simulink model "SOLAR20KW10KW_MOTOR2SWitchesleadacid"  (R2021a)
settings: Solver=VariableStepAuto  StartTime=0.0  StopTime=5  RelTol=1e-3
undefined symbols (not defined in the file): Acid, C_boost, L_boost, Lead
libraries: spsSeriesRLCBranchLib x7, spsVoltageMeasurementLib x3, spsBreakerLib x2, spsCurrentMeasurementLib x2, spsDiodeLib x2, spsIGBTDiodeLib x2, spsPWMGeneratorDCDCLib x2, spsBatteryLib x1, spsMeanLib x1, spsPVArrayLib x1, spspowerguiLib x1
settings Model: Creator=Dell  LastModifiedBy=Dell

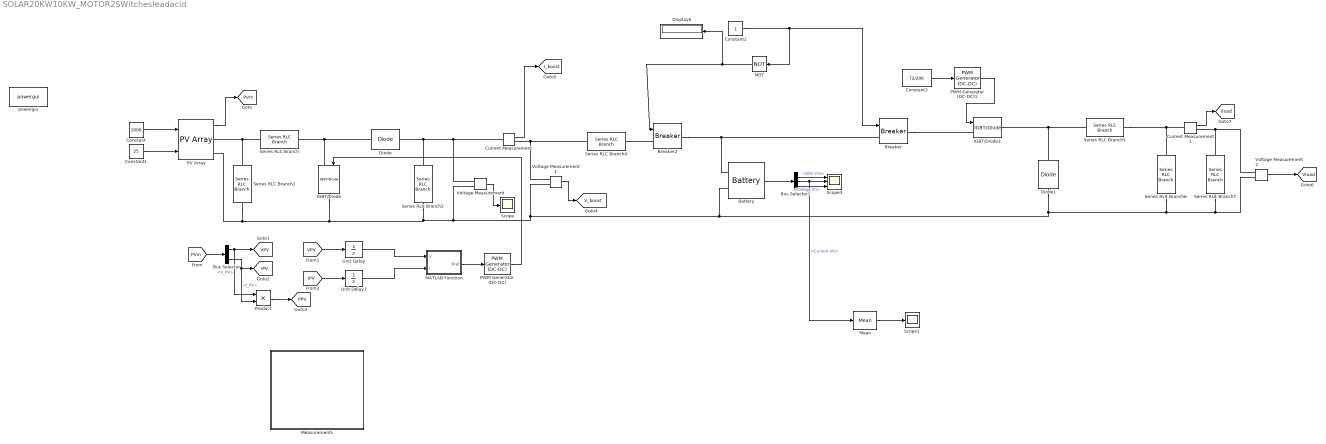
== system SOLAR20KW10KW_MOTOR2SWitchesleadacid ==
  Battery : spsBatteryLib/Battery  BatType=Lead-Acid  ShowTempParam=off  ThermalPreset=no  ShowAgeParam=off  NomV=290  NomQ=150  SOC=50  Batt_Tr=1  PresetModel=on  MaxQ=156.25  MinV=217.5  FullV=315.7566  Dis_rate=30  R=0.019333  Normal_OP=46.5417  expZone="[295.2467           0.5]"  current=[6.5 13 32.5]  Units=Time  Tci=20  NomT=20  T2=-30  MaxQ2=4.8  FullV2=7.1  Normal_OP2=5.655  expZone2="[6.58           1]"  Rca=0.6  ti=2000  Dp=0  Neq0=0  Tsim=1e6  Ta1=25  Qeol=5.4*0.9  Reol=0.013333*1.2  Char_age=[2.3478, 3]  Dis_age=[2.3478, 10]  N1=1500  N2=10500  N3=1000  N4=1400  Ta2=45  N5=950
  Breaker : spsBreakerLib/Breaker  InitialState=0  SwitchingTimes=[3]  External=on  BreakerResistance=0.01  SnubberResistance=1e6  SnubberCapacitance=inf  Measurements=None  MoreParameters=on  NoBreakLoop=off
      settings: SourceProductBaseCode=PS
  Breaker2 : spsBreakerLib/Breaker  InitialState=0  SwitchingTimes=[3]  External=on  BreakerResistance=0.01  SnubberResistance=1e6  SnubberCapacitance=inf  Measurements=None  MoreParameters=on  NoBreakLoop=off
      settings: SourceProductBaseCode=PS
  Bus Selector : BusSelector  OutputSignals=V_PV,I_PV
  Bus Selector1 : BusSelector  OutputSignals=SOC (%),Current (A),Voltage (V)
  Constant : Constant  Value=1000
  Constant1 : Constant  Value=25
  Constant2 : Constant
  Constant3 : Constant  Value=72/290
  Current Measurement : spsCurrentMeasurementLib/Current Measurement  PhasorSimulation=off  OutputType=Complex  PSBequivalent=0
  Current Measurement1 : spsCurrentMeasurementLib/Current Measurement  PhasorSimulation=off  OutputType=Complex  PSBequivalent=0
  Diode : spsDiodeLib/Diode  Ron=0.001  Lon=0  Vf=0.8  IC=0  UseSnubber=0  Rs=500  Cs=250e-9  Measurements=off
  Diode1 : spsDiodeLib/Diode  Ron=0.001  Lon=0  Vf=0.8  IC=0  UseSnubber=0  Rs=500  Cs=250e-9  Measurements=off
  Display6 : Display
  IGBT/Diode : spsIGBTDiodeLib/IGBT//Diode  Ron=1e-3  Rs=1e5  Cs=inf  Measurements=off
  IGBT/Diode1 : spsIGBTDiodeLib/IGBT//Diode  Ron=1e-3  Rs=1e5  Cs=inf  Measurements=off
  MATLAB Function : MATLAB Function  TreatAsAtomicUnit=on
  Mean : spsMeanLib/Mean  Freq=60  Vinit=0  Ts=0
  Measurements : Subsystem
  NOT : Logic  Operator=NOT  IconShape=distinctive  AllPortsSameDT=off  OutDataTypeStr=boolean
  PV Array : spsPVArrayLib/PV Array  Npar=9  Nser=7  PlotType=array @ 1000 W/m2 & specified temperatures  S_vec="[ 1000  500  100 ]"  Temp_C_vec="[ 45 25  ]"  ModuleName=User-defined  PlotWhenSelected=off  Pm=315  Ncell=72  Voc=45.8  Isc=8.92  Vm=37.5  Im=8.4  beta_Voc_pc=-0.36099  alpha_Isc_pc=0.102  beta_Voc=-0.16533  alpha_Isc=0.0090984  IL=8.9507  I0=3.3278e-10  nI=1.0316  Rsh=368.3938  Rs=0.3143  RobustModel=off  RobustCellTemperature=313.3991  BAL=on  Tc=1e-6  Tfilter=5e-5
  PWM Generator (DC-DC) : spsPWMGeneratorDCDCLib/PWM Generator (DC-DC)  Fsw=5000  Ts=0
  PWM Generator (DC-DC)1 : spsPWMGeneratorDCDCLib/PWM Generator (DC-DC)  Fsw=5000  Ts=0
  Product : Product
  Scope : Scope
  Scope1 : Scope
  Scope3 : Scope  NumInputPorts=3
  Series RLC Branch : spsSeriesRLCBranchLib/Series RLC Branch  LConnTagsString=__new0  RConnTagsString=__new0  BranchType=L  Resistance=1  Inductance=L_boost  SetiL0=off  InitialCurrent=0  Capacitance=1e-6  Setx0=off  InitialVoltage=0  Measurements=None
  Series RLC Branch1 : spsSeriesRLCBranchLib/Series RLC Branch  LConnTagsString=__new0  RConnTagsString=__new0  BranchType=C  Resistance=1  Inductance=1e-3  SetiL0=off  InitialCurrent=0  Capacitance=1000e-6  Setx0=off  InitialVoltage=0  Measurements=None
  Series RLC Branch2 : spsSeriesRLCBranchLib/Series RLC Branch  LConnTagsString=__new0  RConnTagsString=__new0  BranchType=C  Resistance=1  Inductance=1e-3  SetiL0=off  InitialCurrent=0  Capacitance=C_boost  Setx0=off  InitialVoltage=0  Measurements=None
  Series RLC Branch4 : spsSeriesRLCBranchLib/Series RLC Branch  LConnTagsString=__new0  RConnTagsString=__new0  BranchType=L  Resistance=1  Inductance=1e-3  SetiL0=off  InitialCurrent=0  Capacitance=1e-6  Setx0=off  InitialVoltage=0  Measurements=None
  Series RLC Branch5 : spsSeriesRLCBranchLib/Series RLC Branch  LConnTagsString=__new0  RConnTagsString=__new0  BranchType=L  Resistance=1  Inductance=0.0078  SetiL0=off  InitialCurrent=0  Capacitance=1e-6  Setx0=off  InitialVoltage=0  Measurements=None
  Series RLC Branch6 : spsSeriesRLCBranchLib/Series RLC Branch  LConnTagsString=__new0  RConnTagsString=__new0  BranchType=RC  Resistance=10e-3  Inductance=1e-3  SetiL0=off  InitialCurrent=0  Capacitance=4.8225e-05  Setx0=off  InitialVoltage=0  Measurements=None
  Series RLC Branch7 : spsSeriesRLCBranchLib/Series RLC Branch  LConnTagsString=__new0  RConnTagsString=__new0  BranchType=R  Resistance=0.5184  Inductance=1e-3  SetiL0=off  InitialCurrent=0  Capacitance=1e-6  Setx0=off  InitialVoltage=0  Measurements=None
  Unit Delay : UnitDelay  SampleTime=-1  HasFrameUpgradeWarning=on
  Unit Delay1 : UnitDelay  SampleTime=-1  HasFrameUpgradeWarning=on
  Voltage Measurement : spsVoltageMeasurementLib/Voltage Measurement  PhasorSimulation=off  OutputType=Complex  PSBequivalent=0
  Voltage Measurement1 : spsVoltageMeasurementLib/Voltage Measurement  PhasorSimulation=off  OutputType=Complex  PSBequivalent=0
  Voltage Measurement2 : spsVoltageMeasurementLib/Voltage Measurement  PhasorSimulation=off  OutputType=Complex  PSBequivalent=0
  powergui : spspowerguiLib/powergui  Priority=1  SimulationMode=Continuous  SampleTime=50e-6  frequency=60  Iterations=50  frequencyindice=0  Pbase=100e6  ErrMax=1e-4  UnitsV=kV  UnitsW=MW  buscounter=0  FunctionMessages=off  echomessages=off  EnableUseOfTLC=off  CurrentSourceSwitches=off  DisableSnubberDevices=off  DisableRonSwitches=off  DisableVfSwitches=off  DisplayEquations=off  AutomaticDiscreteSolvers=off  SolverType=Tustin/Backward Euler (TBE)  Interpol=off  ExternalGateDelay=off  methode=off  Ts=100  x0status=blocks  SPID=on  SwTol=0  HookPort=off  NonlinearTolerance=1e-4  nMaxIteration=100  ContinueOnMaxIteration=off  RestoreLinks=warning  ResistiveCurrentMeasurement=off  Frange=[0:2:500]  Ylog=off  Xlog=on  ShowGrid=off  save=off  variable=ZData  structure=0  ZoomFFT=off  StartTime=0.0  cycles=1  DisplayStyle=1  fundamental=60  FreqAxis=off  MaxFrequency=1000  frequencyindicesteady=1  RmsSteady=1  display=off
  tag scope: IPV=global, I_boost=global, Iload=global, PPV=global, PVm=global, VPV=global, V_boost=global, Vload=global
  wires:
  Constant/1 -> PV Array/1
  Constant1/1 -> PV Array/2
  PV Array/1 -> [PVm]
  [PVm] -> Bus Selector/1
  Bus Selector/1 -> [VPV], Product/1  "<V_PV>"
  Bus Selector/2 -> Product/2, [IPV]  "<I_PV>"
  [VPV] -> Unit Delay/1
  [IPV] -> Unit Delay1/1
  Unit Delay/1 -> MATLAB Function/1(V)
  Unit Delay1/1 -> MATLAB Function/2(I)
  MATLAB Function/1(Dref) -> PWM Generator (DC-DC)/1
  PWM Generator (DC-DC)/1 -> IGBT/Diode/1
  Voltage Measurement/1 -> Scope/1
  Current Measurement/1 -> [I_boost]
  Product/1 -> [PPV]
  Battery/1 -> Bus Selector1/1
  Bus Selector1/1 -> Scope3/1  "<SOC (%)>"
  Bus Selector1/2 -> Mean/1, Scope3/2  "<Current (A)>"
  Bus Selector1/3 -> Scope3/3  "<Voltage (V)>"
  Constant2/1 -> NOT/1, Breaker/1
  Voltage Measurement2/1 -> [Vload]
  PWM Generator (DC-DC)1/1 -> IGBT/Diode1/1
  Constant3/1 -> PWM Generator (DC-DC)1/1
  Voltage Measurement1/1 -> [V_boost]
  NOT/1 -> Display6/1, Breaker2/1
  Current Measurement1/1 -> [Iload]
  Mean/1 -> Scope1/1
  connections:
  Series RLC Branch/LConn1 -- Series RLC Branch1/LConn1 -- PV Array/RConn1
  IGBT/Diode/LConn1 -- Series RLC Branch/RConn1 -- Diode/LConn1
  Series RLC Branch2/LConn1 -- Current Measurement/LConn1 -- Voltage Measurement/LConn1 -- Diode/RConn1
  Voltage Measurement1/LConn1 -- Series RLC Branch4/LConn1 -- Current Measurement/RConn1
  Breaker/LConn1 -- Battery/LConn1 -- Breaker2/RConn1
  Breaker/RConn1 -- IGBT/Diode1/LConn1
  Series RLC Branch5/LConn1 -- Diode1/RConn1 -- IGBT/Diode1/RConn1
  Voltage Measurement2/LConn1 -- Series RLC Branch7/LConn1 -- Current Measurement1/RConn1
  Series RLC Branch5/RConn1 -- Series RLC Branch6/LConn1 -- Current Measurement1/LConn1
  Diode1/LConn1 -- Series RLC Branch1/RConn1 -- PV Array/RConn2 -- IGBT/Diode/RConn1 -- Series RLC Branch2/RConn1 -- Voltage Measurement/LConn2 -- Voltage Measurement1/LConn2 -- Battery/LConn2 -- Series RLC Branch7/RConn1 -- Voltage Measurement2/LConn2 -- Series RLC Branch6/RConn1
  Breaker2/LConn1 -- Series RLC Branch4/RConn1

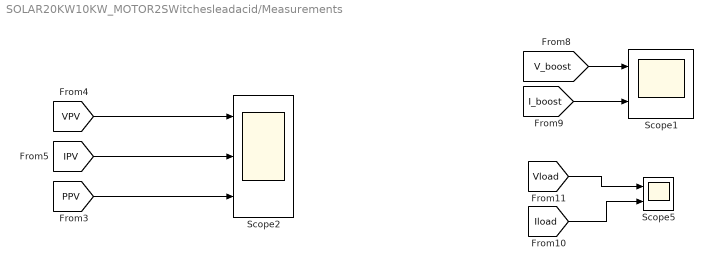
== system SOLAR20KW10KW_MOTOR2SWitchesleadacid/Measurements ==
  Scope1 : Scope  NumInputPorts=2
  Scope2 : Scope  NumInputPorts=3
  Scope5 : Scope  NumInputPorts=2
  wires:
  [VPV] -> Scope2/1
  [PPV] -> Scope2/3
  [IPV] -> Scope2/2
  [V_boost] -> Scope1/1
  [Vload] -> Scope5/1
  [Iload] -> Scope5/2
  [I_boost] -> Scope1/2

== matlab function SOLAR20KW10KW_MOTOR2SWitchesleadacid/MATLAB Function ==
  data: V input; Dref output; I input
function Dref=MPPT(V,I)
duty_init = 0.1;
Dmin = 0.1;
Dmax = 0.9;
deldref=0.00008;
persistent Vold Pold Drefold;
if isempty(Vold)
    Vold=0;
    Pold=0;
    Drefold=duty_init;
end
P=V*I;
dV=V-Vold;
dP=P-Pold;
if dP~=0
    if dP<0
        if dV<0
            Dref=Drefold-deldref;
        else
            Dref=Drefold+deldref;
        end
    else
        if dV<0
            Dref=Drefold+deldref;
        else
            Dref=Drefold-deldref;
        end
    end
else
    Dref=Drefold;
end
if Dref>Dmax || Dref<Dmin
    Dref=Drefold;
end
Drefold=Dref;
Pold=P;
Vold=V;
